simulink model "StFilteringLab"  (Simulink 7.6)
settings: Solver=VariableStepDiscrete  SolverMode=SingleTasking  StartTime=0.0  StopTime=4096*FirSamplingPeriod  RelTol=1e-3
PreLoadFcn:
  | clc
  | clear
  | close all
  | FilterOrder = 34;
  | InputBitWidth = 12;
  | CoefBitWidth = 14;
  | coef_max = 2^(CoefBitWidth - 1) - 1;
  | coef_min = -2^(CoefBitWidth - 1);
  | LowPassFreqBand = [0 0.001045 0.0015 1];
  | LowPassMagnBand = [1 0.975 0.00001 0.00001];
  | 
  | FlCoef_org = firls(FilterOrder,LowPassFreqBand,LowPassMagnBand);
  | w=blackman(FilterOrder + 1);
  | FlCoef_win = FlCoef_org .* w';
  | FlCoef = FlCoef_win;
  | ScalingFactor = max(coef_max/max(FlCoef), coef_min/min(FlCoef));
  | 
  | FpCoef = fix(ScalingFactor * FlCoef);
  | 
  | plot(FpCoef,'o');
  | title('Coefficient Value');
  | ImpulseData = zeros(1,1000);
  | ImpulseData(1) = 100;
  | h = conv(ImpulseData,FpCoef);
  | fftplot(h);
  | title('Frequency response');
  | FirSamplingPeriod=1;
InitFcn:
  | %% DSPBuilder Start
  | alt_dspbuilder_update_model(bdroot)
  | %% DSPBuilder End
StopFcn:
  | plot_fft(adder_result_sim, 'Frequency Response - Unfiltered Data', 8e7)
  |  plot_fft(fir_result_sim, 'Frequency Response - Filtered Data', 8e7)
values from neighbouring files (symbols this model uses):
  data = data(1:N)    [fftplot.m]
undefined symbols (not defined in the file or in its folder): filter_lib, lp_filter, Pin_AB15, Pin_AB6, Pin_AC14, Pin_AC19, Pin_AD14, Pin_AD18, Pin_AE3, Pin_AF25, Pin_AG23, Pin_G20, Pin_G3, Pin_G4, Pin_H3, Pin_H4, Pin_J5, Pin_J6, Pin_K1, Pin_K2, Pin_L1, Pin_L2, Pin_L3, Pin_L4, Pin_M7, Pin_M8, Pin_N3, Pin_N4, Pin_P1, Pin_P2, Pin_R3, Pin_R4, Pin_R6, Pin_R7, Pin_T3, Pin_T4, Pin_V3, Pin_V4, sin_gen
libraries: allblocks_alteradspbuilder2 x68, Cyclone_III_EP3C120_alteradspbuilder2 x5
settings Model: Creator=akarapet  LastModifiedBy=akarapet
settings DataIOCC: SignalLoggingName=sigsOut
settings OptimizationCC: InlineInvariantSignals=on  InitFltsAndDblsToZero=on
settings DebuggingCC: SaveWithParameterizedLinksMsg=none  SignalResolutionControl=TryResolveAllWithWarning  SolverPrmCheckMsg=none  MultiTaskDSMMsg=warning  MultiTaskCondExecSysMsg=none  StrictBusMsg=None
settings HardwareCC: TargetUnknown=on
settings RTWCC: IncludeERTFirstTime=on
settings GRTTargetCC: TargetFcnLib=ansi_tfl_tmw.mat

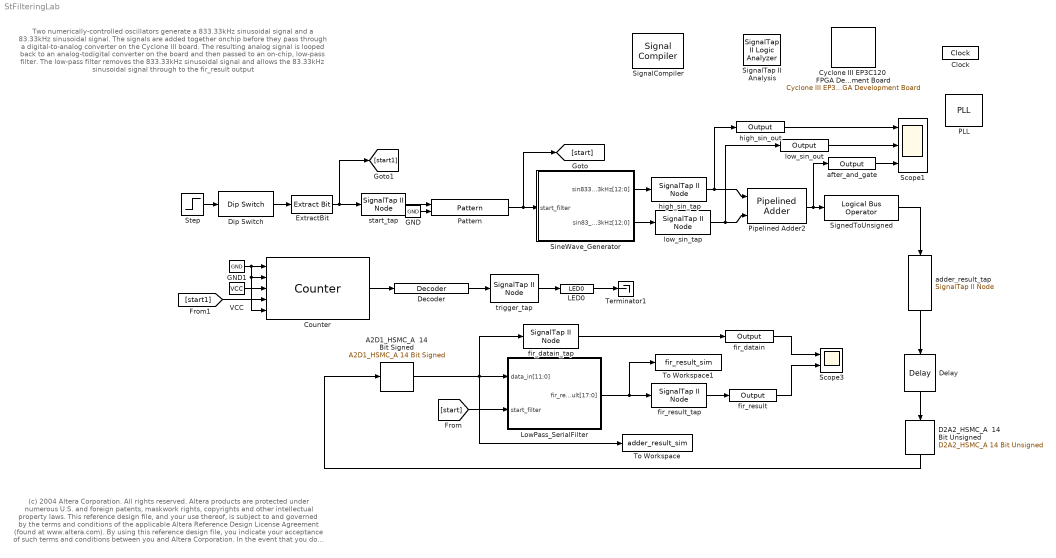
== system StFilteringLab ==
  note: (c) 2004 Altera Corporation. All rights reserved.  Altera products are protected under numerous U.S. and foreign patents, maskwork rights, copyrights and other intellectual property laws.
      | This reference design file, and your use thereof, is subject to and governed by the terms and conditions of the applicable Altera Reference Design License Agreement (found at www.altera.com).
      | By using this reference design file, you indicate your acceptance of such terms and conditions between you and Altera Corporation.
      | In the event that you do not agree with such terms and conditions, you may not use the reference design file and please promptly destroy any copies you have made.
      | This reference design file being provided on an "as-is" basis and as an accommodation and therefore all warranties, representations or guarantees of any kind (whether express, implied or statutory)
      | including, without limitation, warranties of merchantability, non-infringement, or fitness for a particular purpose, are specifically disclaimed.
      | By making this reference design file available, Altera expressly does not recommend, suggest or require that this reference design file be used in combination with any other product not provided by Altera
  note: Two numerically-controlled oscillators generate a 833.33kHz  sinusoidal
      | signal and a 83.33kHz sinusoidal signal. The signals are added together onchip
      | before they pass through a digital-to-analog converter on the Cyclone III board.
      | The resulting analog signal is looped back to an analog-todigital
      | converter on the board and then passed to an on-chip, low-pass
      | filter. The low-pass filter removes the 833.33kHz sinusoidal signal and
      | allows the 83.33kHz sinusoidal signal
      | through to the fir_result output
  A2D1_HSMC_A  14 Bit Signed : Cyclone_III_EP3C120_alteradspbuilder2/A2D1_HSMC_A 14 Bit Signed  iofile=/data/akarapet/qshell_linux64_test/p4/dsp_builder/dsp_builder2/Documentation/DesignExamples/Demos/Filters/FilteringLab/Stap/tb_StFilteringLab/StFilteringLab_A2D1%5FHSMC%5FA+%0A14+Bit+Signed.salt  externalType=Inferred  SpecifyClock=off  location=Pin_P1,Pin_P2,Pin_M7,Pin_M8,Pin_R4,Pin_R3,Pin_T3,Pin_T4,Pin_V3,Pin_V4,Pin_R6,Pin_R7,Pin_AE3,Pin_AB6
  Clock : allblocks_alteradspbuilder2/Clock  ClockPeriod=10  ClockPeriodUnit=ns  SampleTime=1  ResetLatency=0  ResetRegisterCascadeDepth=0  SimulationStartCycle=5  PhaseOffset=0  Reset=aclr  ResetType=Active Low  Export=off
  Counter : allblocks_alteradspbuilder2/Counter  BusType=Signed Integer  bwl=13  bwr=0  use_modulo=on  modulo=2^12 - 1  SpecifyClock=off  direction=Use Direction Port (updown)  use_sload=on  use_sset=off  svalue=1  use_clk_ena=on  use_ena=off  use_sclr=on  pipeline_display=1
  Cyclone III EP3C120  FPGA Development Board : Cyclone_III_EP3C120_alteradspbuilder2/Cyclone III EP3C120 FPGA Development Board  ClockPinIn=Pin_AH15  GlobalResetPin=Pin_T21  device=EP3C120F780C7
  D2A2_HSMC_A  14 Bit Unsigned : Cyclone_III_EP3C120_alteradspbuilder2/D2A2_HSMC_A 14 Bit Unsigned  iofile=/data/akarapet/qshell_linux64_test/p4/dsp_builder/dsp_builder2/Documentation/DesignExamples/Demos/Filters/FilteringLab/Stap/tb_StFilteringLab/StFilteringLab_D2A2%5FHSMC%5FA+%0A14+Bit+Unsigned.capture  externalType=Inferred  location=Pin_G3,Pin_G4,Pin_H3,Pin_H4,Pin_J5,Pin_J6,Pin_K1,Pin_K2,Pin_L1,Pin_L2,Pin_L3,Pin_L4,Pin_N3,Pin_N4
  Decoder : allblocks_alteradspbuilder2/Decoder  BusType=Signed Integer  bwl=13  bwr=0  registered=off  pipeline_display=0  value=1000
  Delay : allblocks_alteradspbuilder2/Delay  pipeline=1  pipeline_display=1  ClockPhase=1  use_ena=off  use_sclr=off  allowFloatingPointOverride=on  logOutputs=off  logFile=/data/akarapet/qshell_linux64_test/p4/dsp_builder/dsp_builder2/Documentation/DesignExamples/Demos/Filters/FilteringLab/Stap/tb_StFilteringLab/StFilteringLab_Delay.fixedpointlog  use_init=off  reset_value=1
  Dip Switch : Cyclone_III_EP3C120_alteradspbuilder2/Dip Switch  iofile=/data/akarapet/qshell_linux64_test/p4/dsp_builder/dsp_builder2/Documentation/DesignExamples/Demos/Filters/FilteringLab/Stap/tb_StFilteringLab/StFilteringLab_Dip+Switch.salt  externalType=Inferred  SpecifyClock=off  location=Pin_AC14,Pin_AD18,Pin_AG23,Pin_AC19,Pin_AD14,Pin_G20,Pin_AB15,Pin_AF25
  ExtractBit : allblocks_alteradspbuilder2/Extract Bit  BusType=Signed Fractional  bwl=8  bwr=0  bitToSelect=0  pipeline_display=0
  GND : allblocks_alteradspbuilder2/GND  SpecifyClock=off
  GND1 : allblocks_alteradspbuilder2/GND  SpecifyClock=off
  LED0 : Cyclone_III_EP3C120_alteradspbuilder2/LED0  iofile=/data/akarapet/qshell_linux64_test/p4/dsp_builder/dsp_builder2/Documentation/DesignExamples/Demos/Filters/FilteringLab/Stap/tb_StFilteringLab/StFilteringLab_LED0.capture  externalType=Inferred  location=Pin_AD15
  LowPass_SerialFilter : Subsystem  AncestorBlock=filter_lib/lp_filter
      mask Type: SubSystem AlteraBlockSet
  PLL : allblocks_alteradspbuilder2/PLL  clock_mult=[1, 1, 1, 1, 1, 1, 1, 1, 1]  clock_divide=[1, 1, 1, 1, 1, 1, 1, 1, 1]  clock_export=[1, 1, 1, 0, 0, 0, 0, 0, 0]  num_clocks=3  input_clock=Clock  use_base_clock=on
  Pattern : allblocks_alteradspbuilder2/Pattern  Sequence=100000000000  SpecifyClock=off  use_ena=on  use_sclr=on
  Pipelined Adder2 : allblocks_alteradspbuilder2/Pipelined Adder  BusType=Signed Integer  bwl=14  bwr=0  pipeline=1  pipeline_display=1  AddSubDirection=ADD  use_cin=off  use_ovl=off  use_addsub=off  use_ena=off  use_aclr=off  or_aclr_inputs=on
  Scope1 : Scope  NumInputPorts=3
      settings: YMin=-5~-5~-5  YMax=5~5~5  SaveName=ScopeData3
  Scope3 : Scope  NumInputPorts=2
      settings: YMin=-5~-5  YMax=5~5
  SignalCompiler : allblocks_alteradspbuilder2/Signal Compiler  DeviceFamily=Cyclone III  DeviceName=EP3C120F780C7  EnableSignalTap=on  SignalTapDepth=2048  UseBoardBlock=on  StpUseDefaultClock=on  StpClock=Clock  ExportDir=<binary blob, 123 chars, not shown>
  SignalTap II Analysis : allblocks_alteradspbuilder2/SignalTap II Logic Analyzer
  SignedToUnsigned : allblocks_alteradspbuilder2/Logical Bus Operator  BusType=Signed Fractional  bwl=14  bwr=0  LogicalOp_text=XOR  mask_value_num=8192  shift_amount=3  force_sign_ext=off  pipeline_display=0
  SineWave_Generator : Subsystem  AncestorBlock=filter_lib/sin_gen
      mask Type: SubSystem AlteraBlockSet
  Step : Step  SampleTime=FirSamplingPeriod
  Terminator1 : Terminator
  To Workspace : ToWorkspace  VariableName=adder_result_sim  SampleTime=FirSamplingPeriod  SaveFormat=Array
  To Workspace1 : ToWorkspace  VariableName=fir_result_sim  SampleTime=FirSamplingPeriod  SaveFormat=Array
  VCC : allblocks_alteradspbuilder2/VCC  SpecifyClock=off
  adder_result_tap : allblocks_alteradspbuilder2/SignalTap II Node  id=0
  after_and_gate : allblocks_alteradspbuilder2/Output  iofile=/data/akarapet/qshell_linux64_test/p4/dsp_builder/dsp_builder2/Documentation/DesignExamples/Demos/Filters/FilteringLab/Stap/tb_StFilteringLab/StFilteringLab_after%5Fand%5Fgate.capture  BusType=Signed Integer  bwl=14  bwr=0  externalType=Inferred  PORTTYPE=Output  allowFloatingPointOverride=on  logOutputs=off
  fir_datain : allblocks_alteradspbuilder2/Output  iofile=/data/akarapet/qshell_linux64_test/p4/dsp_builder/dsp_builder2/Documentation/DesignExamples/Demos/Filters/FilteringLab/Stap/tb_StFilteringLab/StFilteringLab_fir%5Fdatain.capture  BusType=Signed Integer  bwl=12  bwr=0  externalType=Inferred  PORTTYPE=Output  allowFloatingPointOverride=on  logOutputs=off
  fir_datain_tap : allblocks_alteradspbuilder2/SignalTap II Node  id=1
  fir_result : allblocks_alteradspbuilder2/Output  iofile=/data/akarapet/qshell_linux64_test/p4/dsp_builder/dsp_builder2/Documentation/DesignExamples/Demos/Filters/FilteringLab/Stap/tb_StFilteringLab/StFilteringLab_fir%5Fresult.capture  BusType=Signed Integer  bwl=18  bwr=0  externalType=Inferred  PORTTYPE=Output  allowFloatingPointOverride=on  logOutputs=off
  fir_result_tap : allblocks_alteradspbuilder2/SignalTap II Node  id=2
  high_sin_out : allblocks_alteradspbuilder2/Output  iofile=/data/akarapet/qshell_linux64_test/p4/dsp_builder/dsp_builder2/Documentation/DesignExamples/Demos/Filters/FilteringLab/Stap/tb_StFilteringLab/StFilteringLab_high%5Fsin%5Fout.capture  BusType=Signed Integer  bwl=13  bwr=0  externalType=Inferred  PORTTYPE=Output  allowFloatingPointOverride=on  logOutputs=off
  high_sin_tap : allblocks_alteradspbuilder2/SignalTap II Node  id=3
  low_sin_out : allblocks_alteradspbuilder2/Output  iofile=/data/akarapet/qshell_linux64_test/p4/dsp_builder/dsp_builder2/Documentation/DesignExamples/Demos/Filters/FilteringLab/Stap/tb_StFilteringLab/StFilteringLab_low%5Fsin%5Fout.capture  BusType=Signed Integer  bwl=13  bwr=0  externalType=Inferred  PORTTYPE=Output  allowFloatingPointOverride=on  logOutputs=off
  low_sin_tap : allblocks_alteradspbuilder2/SignalTap II Node  id=4
  start_tap : allblocks_alteradspbuilder2/SignalTap II Node  id=5
  trigger_tap : allblocks_alteradspbuilder2/SignalTap II Node  id=6
  wires:
  LowPass_SerialFilter/1(fir_result[17:0]) -> To Workspace1/1, fir_result_tap/1
  ExtractBit/1 -> start_tap/1, [start1]
  Step/1 -> Dip Switch/1
  GND/1 -> Pattern/2
  A2D1_HSMC_A  14 Bit Signed/1 -> LowPass_SerialFilter/1(data_in[11:0]), To Workspace/1, fir_datain_tap/1
  [start] -> LowPass_SerialFilter/2(start_filter)
  SignedToUnsigned/1 -> adder_result_tap/1
  SineWave_Generator/1(sin833_33kHz[12:0]) -> high_sin_tap/1
  SineWave_Generator/2(sin83_33kHz[12:0]) -> low_sin_tap/1
  adder_result_tap/1 -> Delay/1
  fir_result_tap/1 -> fir_result/1
  fir_result/1 -> Scope3/2
  Dip Switch/1 -> ExtractBit/1
  start_tap/1 -> Pattern/1
  high_sin_tap/1 -> Pipelined Adder2/1, high_sin_out/1
  low_sin_tap/1 -> Pipelined Adder2/2, low_sin_out/1
  [start1] -> Counter/4
  Decoder/1 -> trigger_tap/1
  Counter/1 -> Decoder/1
  trigger_tap/1 -> LED0/1
  VCC/1 -> Counter/3
  fir_datain_tap/1 -> fir_datain/1
  fir_datain/1 -> Scope3/1
  Delay/1 -> D2A2_HSMC_A  14 Bit Unsigned/1
  Pipelined Adder2/1 -> SignedToUnsigned/1, after_and_gate/1
  GND1/1 -> Counter/1, Counter/2, Counter/5
  Pattern/1 -> [start], SineWave_Generator/1(start_filter)
  high_sin_out/1 -> Scope1/1
  low_sin_out/1 -> Scope1/2
  after_and_gate/1 -> Scope1/3
  D2A2_HSMC_A  14 Bit Unsigned/1 -> A2D1_HSMC_A  14 Bit Signed/1
  LED0/1 -> Terminator1/1

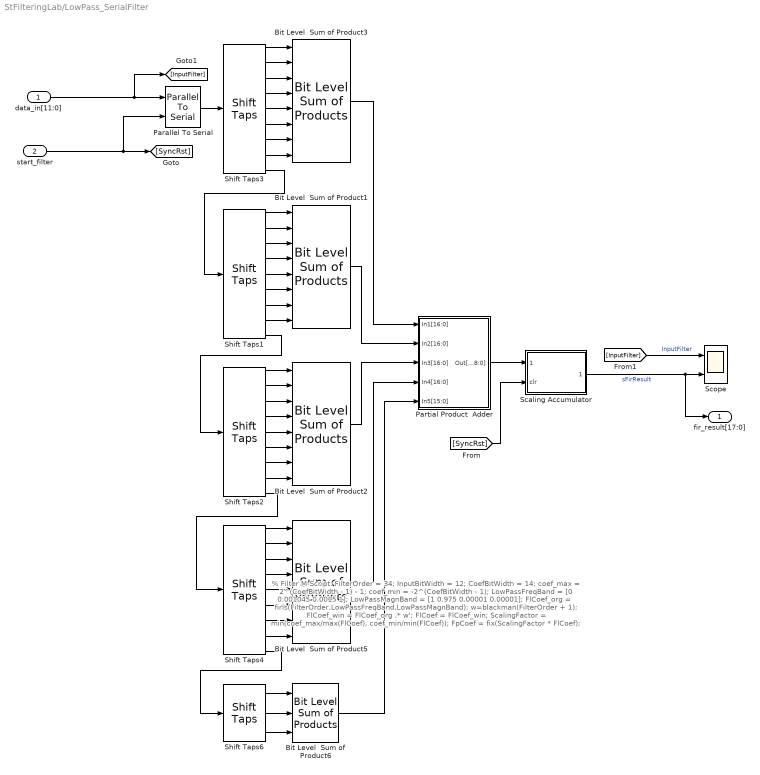
== system StFilteringLab/LowPass_SerialFilter ==
  note: % Filter M-Script:
      | FilterOrder = 34;
      | InputBitWidth = 12;
      | CoefBitWidth = 14;
      | coef_max = 2^(CoefBitWidth - 1) - 1;
      | coef_min = -2^(CoefBitWidth - 1);
      | LowPassFreqBand = [0 0.001045 0.0015 1];
      | LowPassMagnBand = [1 0.975 0.00001 0.00001];
      | FlCoef_org = firls(FilterOrder,LowPassFreqBand,LowPassMagnBand);
      | w=blackman(FilterOrder + 1);
      | FlCoef_win = FlCoef_org .* w';
      | FlCoef = FlCoef_win;
      | ScalingFactor = min(coef_max/max(FlCoef), coef_min/min(FlCoef));
      | FpCoef = fix(ScalingFactor * FlCoef);
  data_in[11:0] : Inport
  start_filter : Inport  Port=2
  Bit Level  Sum of Product1 : allblocks_alteradspbuilder2/Bit Level Sum of Products  number_of_coefficients=8  BusType=Signed Integer  bwl=14  bwr=0  coefficients=[FpCoef(9:16)]  register_inputs=off  pipeline_display=0  use_ena=off  use_sclr=off  allowFloatingPointOverride=on  logOutputs=off  logFile=/data/akarapet/qshell_linux64_test/p4/dsp_builder/dsp_builder2/Documentation/DesignExamples/Demos/Filters/FilteringLab/Stap/tb_StFilteringLab/StFilteringLab_LowPass%5FSerialFilter_Bit+Level+%0ASum+of+Product1.fixedpointlog
  Bit Level  Sum of Product2 : allblocks_alteradspbuilder2/Bit Level Sum of Products  number_of_coefficients=8  BusType=Signed Integer  bwl=14  bwr=0  coefficients=[FpCoef(17:24)]  register_inputs=off  pipeline_display=0  use_ena=off  use_sclr=off  allowFloatingPointOverride=on  logOutputs=off  logFile=/data/akarapet/qshell_linux64_test/p4/dsp_builder/dsp_builder2/Documentation/DesignExamples/Demos/Filters/FilteringLab/Stap/tb_StFilteringLab/StFilteringLab_LowPass%5FSerialFilter_Bit+Level+%0ASum+of+Product2.fixedpointlog
  Bit Level  Sum of Product3 : allblocks_alteradspbuilder2/Bit Level Sum of Products  number_of_coefficients=8  BusType=Signed Integer  bwl=14  bwr=0  coefficients=[FpCoef(1:8)]  register_inputs=off  pipeline_display=0  use_ena=off  use_sclr=off  allowFloatingPointOverride=on  logOutputs=off  logFile=/data/akarapet/qshell_linux64_test/p4/dsp_builder/dsp_builder2/Documentation/DesignExamples/Demos/Filters/FilteringLab/Stap/tb_StFilteringLab/StFilteringLab_LowPass%5FSerialFilter_Bit+Level+%0ASum+of+Product3.fixedpointlog
  Bit Level  Sum of Product5 : allblocks_alteradspbuilder2/Bit Level Sum of Products  number_of_coefficients=8  BusType=Signed Integer  bwl=14  bwr=0  coefficients=[FpCoef(25:32)]  register_inputs=off  pipeline_display=0  use_ena=off  use_sclr=off  allowFloatingPointOverride=on  logOutputs=off  logFile=/data/akarapet/qshell_linux64_test/p4/dsp_builder/dsp_builder2/Documentation/DesignExamples/Demos/Filters/FilteringLab/Stap/tb_StFilteringLab/StFilteringLab_LowPass%5FSerialFilter_Bit+Level+%0ASum+of+Product5.fixedpointlog
  Bit Level  Sum of Product6 : allblocks_alteradspbuilder2/Bit Level Sum of Products  number_of_coefficients=3  BusType=Signed Integer  bwl=14  bwr=0  coefficients=[FpCoef(33:35)]  register_inputs=off  pipeline_display=0  use_ena=off  use_sclr=off  allowFloatingPointOverride=on  logOutputs=off  logFile=/data/akarapet/qshell_linux64_test/p4/dsp_builder/dsp_builder2/Documentation/DesignExamples/Demos/Filters/FilteringLab/Stap/tb_StFilteringLab/StFilteringLab_LowPass%5FSerialFilter_Bit+Level+%0ASum+of+Product6.fixedpointlog
  Parallel To Serial : allblocks_alteradspbuilder2/Parallel To Serial  BusType=Signed Integer  bwl=12  bwr=0  msbfirsttext=LSB First  msbfirst=0  repeatlastbit=on  use_ena=off  use_sclr=off
  Partial Product  Adder : Subsystem  AncestorBlock=ALTELINK/AltLab/HDL SubSystem
      mask Type: SubSystem AlteraBlockSet
  Scaling Accumulator : Subsystem  AncestorBlock=ALTELINK/AltLab/HDL SubSystem
      mask Type: SubSystem AlteraBlockSet
  Scope : Scope  NumInputPorts=2
      settings: YMin=-125~-25  YMax=125~25
  Shift Taps1 : allblocks_alteradspbuilder2/Shift Taps  number_of_taps=8  tap_distance=12  use_shiftout=on  use_ena=off  use_sclr=off  use_dedicated_circuitry=on  ram_type=AUTO  allowFloatingPointOverride=on  logOutputs=off  logFile=/data/akarapet/qshell_linux64_test/p4/dsp_builder/dsp_builder2/Documentation/DesignExamples/Demos/Filters/FilteringLab/Stap/tb_StFilteringLab/StFilteringLab_LowPass%5FSerialFilter_Shift+Taps1%3A%3At.fixedpointlog,/data/akarapet/qshell_linux64_test/p4/dsp_builder/dsp_builder2/Documentation/DesignExamples/Demos/Filters/FilteringLab/Stap/tb_StFilteringLab/StFilteringLab_LowPass%5FSerialFilter_Shift+Taps1%3A%3At.fixedpointlog,/data/akarapet/qshell_linux64_test/p4/dsp_builder/dsp_builder2/Documentation/DesignExamples/Demos/Filters/FilteringLab/Stap/tb_StFilteringLab/StFilteringLab_LowPass%5FSerialFilter_Shift+Taps1%3A%3At.fixedpointlog,/data/akarapet/qshell_linux64_test/p4/dsp_builder/dsp_builder2/Documentation/DesignExamples/Demos/Filters/FilteringLab/Stap/tb_StFilteringLab/StFilteringLab_LowPass%5FSerialFilter_Shift+Taps1%3A%3At.fixedpointlog,/data/akarapet/qshell_linux64_test/p4/dsp_builder/dsp_builder2/Documentation/DesignExamples/Demos/Filters/FilteringLab/Stap/tb_StFilteringLab/StFilteringLab_LowPass%5FSerialFilter_Shift+Taps1%3A%3At.fixedpointlog,/data/akarapet/qshell_linux64_test/p4/dsp_builder/dsp_builder2/Documentation/DesignExamples/Demos/Filters/FilteringLab/Stap/tb_StFilteringLab/StFilteringLab_LowPass%5FSerialFilter_Shift+Taps1%3A%3At.fixedpointlog,/data/akarapet/qshell_linux64_test/p4/dsp_builder/dsp_builder2/Documentation/DesignExamples/Demos/Filters/FilteringLab/Stap/tb_StFilteringLab/StFilteringLab_LowPass%5FSerialFilter_Shift+Taps1%3A%3At.fixedpointlog,/data/akarapet/qshell_linux64_test/p4/dsp_builder/dsp_builder2/Documentation/DesignExamples/Demos/Filters/FilteringLab/Stap/tb_StFilteringLab/StFilteringLab_LowPass%5FSerialFilter_Shift+Taps1%3A%3At.fixedpointlog,/data/akarapet/qshell_linux64_test/p4/dsp_builder/dsp_builder2/Documentation/DesignExamples/Demos/Filters/FilteringLab/Stap/tb_StFilteringLab/StFilteringLab_LowPass%5FSerialFilter_Shift+Taps1%3A%3Ashiftout.fixedpointlog,
  Shift Taps2 : allblocks_alteradspbuilder2/Shift Taps  number_of_taps=8  tap_distance=12  use_shiftout=on  use_ena=off  use_sclr=off  use_dedicated_circuitry=on  ram_type=AUTO  allowFloatingPointOverride=on  logOutputs=off  logFile=/data/akarapet/qshell_linux64_test/p4/dsp_builder/dsp_builder2/Documentation/DesignExamples/Demos/Filters/FilteringLab/Stap/tb_StFilteringLab/StFilteringLab_LowPass%5FSerialFilter_Shift+Taps2%3A%3At.fixedpointlog,/data/akarapet/qshell_linux64_test/p4/dsp_builder/dsp_builder2/Documentation/DesignExamples/Demos/Filters/FilteringLab/Stap/tb_StFilteringLab/StFilteringLab_LowPass%5FSerialFilter_Shift+Taps2%3A%3At.fixedpointlog,/data/akarapet/qshell_linux64_test/p4/dsp_builder/dsp_builder2/Documentation/DesignExamples/Demos/Filters/FilteringLab/Stap/tb_StFilteringLab/StFilteringLab_LowPass%5FSerialFilter_Shift+Taps2%3A%3At.fixedpointlog,/data/akarapet/qshell_linux64_test/p4/dsp_builder/dsp_builder2/Documentation/DesignExamples/Demos/Filters/FilteringLab/Stap/tb_StFilteringLab/StFilteringLab_LowPass%5FSerialFilter_Shift+Taps2%3A%3At.fixedpointlog,/data/akarapet/qshell_linux64_test/p4/dsp_builder/dsp_builder2/Documentation/DesignExamples/Demos/Filters/FilteringLab/Stap/tb_StFilteringLab/StFilteringLab_LowPass%5FSerialFilter_Shift+Taps2%3A%3At.fixedpointlog,/data/akarapet/qshell_linux64_test/p4/dsp_builder/dsp_builder2/Documentation/DesignExamples/Demos/Filters/FilteringLab/Stap/tb_StFilteringLab/StFilteringLab_LowPass%5FSerialFilter_Shift+Taps2%3A%3At.fixedpointlog,/data/akarapet/qshell_linux64_test/p4/dsp_builder/dsp_builder2/Documentation/DesignExamples/Demos/Filters/FilteringLab/Stap/tb_StFilteringLab/StFilteringLab_LowPass%5FSerialFilter_Shift+Taps2%3A%3At.fixedpointlog,/data/akarapet/qshell_linux64_test/p4/dsp_builder/dsp_builder2/Documentation/DesignExamples/Demos/Filters/FilteringLab/Stap/tb_StFilteringLab/StFilteringLab_LowPass%5FSerialFilter_Shift+Taps2%3A%3At.fixedpointlog,/data/akarapet/qshell_linux64_test/p4/dsp_builder/dsp_builder2/Documentation/DesignExamples/Demos/Filters/FilteringLab/Stap/tb_StFilteringLab/StFilteringLab_LowPass%5FSerialFilter_Shift+Taps2%3A%3Ashiftout.fixedpointlog,
  Shift Taps3 : allblocks_alteradspbuilder2/Shift Taps  number_of_taps=8  tap_distance=12  use_shiftout=on  use_ena=off  use_sclr=off  use_dedicated_circuitry=on  ram_type=AUTO  allowFloatingPointOverride=on  logOutputs=off  logFile=/data/akarapet/qshell_linux64_test/p4/dsp_builder/dsp_builder2/Documentation/DesignExamples/Demos/Filters/FilteringLab/Stap/tb_StFilteringLab/StFilteringLab_LowPass%5FSerialFilter_Shift+Taps3%3A%3At.fixedpointlog,/data/akarapet/qshell_linux64_test/p4/dsp_builder/dsp_builder2/Documentation/DesignExamples/Demos/Filters/FilteringLab/Stap/tb_StFilteringLab/StFilteringLab_LowPass%5FSerialFilter_Shift+Taps3%3A%3At.fixedpointlog,/data/akarapet/qshell_linux64_test/p4/dsp_builder/dsp_builder2/Documentation/DesignExamples/Demos/Filters/FilteringLab/Stap/tb_StFilteringLab/StFilteringLab_LowPass%5FSerialFilter_Shift+Taps3%3A%3At.fixedpointlog,/data/akarapet/qshell_linux64_test/p4/dsp_builder/dsp_builder2/Documentation/DesignExamples/Demos/Filters/FilteringLab/Stap/tb_StFilteringLab/StFilteringLab_LowPass%5FSerialFilter_Shift+Taps3%3A%3At.fixedpointlog,/data/akarapet/qshell_linux64_test/p4/dsp_builder/dsp_builder2/Documentation/DesignExamples/Demos/Filters/FilteringLab/Stap/tb_StFilteringLab/StFilteringLab_LowPass%5FSerialFilter_Shift+Taps3%3A%3At.fixedpointlog,/data/akarapet/qshell_linux64_test/p4/dsp_builder/dsp_builder2/Documentation/DesignExamples/Demos/Filters/FilteringLab/Stap/tb_StFilteringLab/StFilteringLab_LowPass%5FSerialFilter_Shift+Taps3%3A%3At.fixedpointlog,/data/akarapet/qshell_linux64_test/p4/dsp_builder/dsp_builder2/Documentation/DesignExamples/Demos/Filters/FilteringLab/Stap/tb_StFilteringLab/StFilteringLab_LowPass%5FSerialFilter_Shift+Taps3%3A%3At.fixedpointlog,/data/akarapet/qshell_linux64_test/p4/dsp_builder/dsp_builder2/Documentation/DesignExamples/Demos/Filters/FilteringLab/Stap/tb_StFilteringLab/StFilteringLab_LowPass%5FSerialFilter_Shift+Taps3%3A%3At.fixedpointlog,/data/akarapet/qshell_linux64_test/p4/dsp_builder/dsp_builder2/Documentation/DesignExamples/Demos/Filters/FilteringLab/Stap/tb_StFilteringLab/StFilteringLab_LowPass%5FSerialFilter_Shift+Taps3%3A%3Ashiftout.fixedpointlog,
  Shift Taps4 : allblocks_alteradspbuilder2/Shift Taps  number_of_taps=8  tap_distance=12  use_shiftout=on  use_ena=off  use_sclr=off  use_dedicated_circuitry=on  ram_type=AUTO  allowFloatingPointOverride=on  logOutputs=off  logFile=/data/akarapet/qshell_linux64_test/p4/dsp_builder/dsp_builder2/Documentation/DesignExamples/Demos/Filters/FilteringLab/Stap/tb_StFilteringLab/StFilteringLab_LowPass%5FSerialFilter_Shift+Taps4%3A%3At.fixedpointlog,/data/akarapet/qshell_linux64_test/p4/dsp_builder/dsp_builder2/Documentation/DesignExamples/Demos/Filters/FilteringLab/Stap/tb_StFilteringLab/StFilteringLab_LowPass%5FSerialFilter_Shift+Taps4%3A%3At.fixedpointlog,/data/akarapet/qshell_linux64_test/p4/dsp_builder/dsp_builder2/Documentation/DesignExamples/Demos/Filters/FilteringLab/Stap/tb_StFilteringLab/StFilteringLab_LowPass%5FSerialFilter_Shift+Taps4%3A%3At.fixedpointlog,/data/akarapet/qshell_linux64_test/p4/dsp_builder/dsp_builder2/Documentation/DesignExamples/Demos/Filters/FilteringLab/Stap/tb_StFilteringLab/StFilteringLab_LowPass%5FSerialFilter_Shift+Taps4%3A%3At.fixedpointlog,/data/akarapet/qshell_linux64_test/p4/dsp_builder/dsp_builder2/Documentation/DesignExamples/Demos/Filters/FilteringLab/Stap/tb_StFilteringLab/StFilteringLab_LowPass%5FSerialFilter_Shift+Taps4%3A%3At.fixedpointlog,/data/akarapet/qshell_linux64_test/p4/dsp_builder/dsp_builder2/Documentation/DesignExamples/Demos/Filters/FilteringLab/Stap/tb_StFilteringLab/StFilteringLab_LowPass%5FSerialFilter_Shift+Taps4%3A%3At.fixedpointlog,/data/akarapet/qshell_linux64_test/p4/dsp_builder/dsp_builder2/Documentation/DesignExamples/Demos/Filters/FilteringLab/Stap/tb_StFilteringLab/StFilteringLab_LowPass%5FSerialFilter_Shift+Taps4%3A%3At.fixedpointlog,/data/akarapet/qshell_linux64_test/p4/dsp_builder/dsp_builder2/Documentation/DesignExamples/Demos/Filters/FilteringLab/Stap/tb_StFilteringLab/StFilteringLab_LowPass%5FSerialFilter_Shift+Taps4%3A%3At.fixedpointlog,/data/akarapet/qshell_linux64_test/p4/dsp_builder/dsp_builder2/Documentation/DesignExamples/Demos/Filters/FilteringLab/Stap/tb_StFilteringLab/StFilteringLab_LowPass%5FSerialFilter_Shift+Taps4%3A%3Ashiftout.fixedpointlog,
  Shift Taps6 : allblocks_alteradspbuilder2/Shift Taps  number_of_taps=3  tap_distance=12  use_shiftout=off  use_ena=off  use_sclr=off  use_dedicated_circuitry=on  ram_type=AUTO  allowFloatingPointOverride=on  logOutputs=off  logFile=/data/akarapet/qshell_linux64_test/p4/dsp_builder/dsp_builder2/Documentation/DesignExamples/Demos/Filters/FilteringLab/Stap/tb_StFilteringLab/StFilteringLab_LowPass%5FSerialFilter_Shift+Taps6%3A%3At.fixedpointlog,/data/akarapet/qshell_linux64_test/p4/dsp_builder/dsp_builder2/Documentation/DesignExamples/Demos/Filters/FilteringLab/Stap/tb_StFilteringLab/StFilteringLab_LowPass%5FSerialFilter_Shift+Taps6%3A%3At.fixedpointlog,/data/akarapet/qshell_linux64_test/p4/dsp_builder/dsp_builder2/Documentation/DesignExamples/Demos/Filters/FilteringLab/Stap/tb_StFilteringLab/StFilteringLab_LowPass%5FSerialFilter_Shift+Taps6%3A%3At.fixedpointlog,
  fir_result[17:0] : Outport
  wires:
  Bit Level  Sum of Product6/1 -> Partial Product  Adder/5(In5[15:0])
  Bit Level  Sum of Product5/1 -> Partial Product  Adder/4(In4[16:0])
  Bit Level  Sum of Product2/1 -> Partial Product  Adder/3(In3[16:0])
  Bit Level  Sum of Product1/1 -> Partial Product  Adder/2(In2[16:0])
  Bit Level  Sum of Product3/1 -> Partial Product  Adder/1(In1[16:0])
  Shift Taps4/8 -> Bit Level  Sum of Product5/8
  Shift Taps4/7 -> Bit Level  Sum of Product5/7
  Shift Taps4/6 -> Bit Level  Sum of Product5/6
  Shift Taps4/5 -> Bit Level  Sum of Product5/5
  Shift Taps4/4 -> Bit Level  Sum of Product5/4
  Shift Taps4/3 -> Bit Level  Sum of Product5/3
  Shift Taps4/2 -> Bit Level  Sum of Product5/2
  Shift Taps4/1 -> Bit Level  Sum of Product5/1
  Shift Taps3/9 -> Shift Taps1/1
  Shift Taps3/8 -> Bit Level  Sum of Product3/8
  Shift Taps3/7 -> Bit Level  Sum of Product3/7
  Shift Taps3/6 -> Bit Level  Sum of Product3/6
  Shift Taps3/5 -> Bit Level  Sum of Product3/5
  Shift Taps3/4 -> Bit Level  Sum of Product3/4
  Shift Taps3/3 -> Bit Level  Sum of Product3/3
  Shift Taps3/2 -> Bit Level  Sum of Product3/2
  Shift Taps3/1 -> Bit Level  Sum of Product3/1
  Scaling Accumulator/1(Out[17:0]) -> fir_result[17:0]/1, Scope/2  "sFirResult"
  [InputFilter] -> Scope/1  "InputFilter"
  data_in[11:0]/1 -> Parallel To Serial/1, [InputFilter]
  Shift Taps2/9 -> Shift Taps4/1
  Shift Taps4/9 -> Shift Taps6/1
  Shift Taps6/3 -> Bit Level  Sum of Product6/3
  Shift Taps6/2 -> Bit Level  Sum of Product6/2
  Shift Taps6/1 -> Bit Level  Sum of Product6/1
  Partial Product  Adder/1(Out[18:0]) -> Scaling Accumulator/1(In[18:0])
  Parallel To Serial/1 -> Shift Taps3/1
  Shift Taps1/9 -> Shift Taps2/1
  Shift Taps2/8 -> Bit Level  Sum of Product2/8
  Shift Taps2/7 -> Bit Level  Sum of Product2/7
  Shift Taps2/6 -> Bit Level  Sum of Product2/6
  Shift Taps2/5 -> Bit Level  Sum of Product2/5
  Shift Taps2/4 -> Bit Level  Sum of Product2/4
  Shift Taps2/3 -> Bit Level  Sum of Product2/3
  Shift Taps2/2 -> Bit Level  Sum of Product2/2
  Shift Taps2/1 -> Bit Level  Sum of Product2/1
  Shift Taps1/8 -> Bit Level  Sum of Product1/8
  Shift Taps1/7 -> Bit Level  Sum of Product1/7
  Shift Taps1/6 -> Bit Level  Sum of Product1/6
  Shift Taps1/5 -> Bit Level  Sum of Product1/5
  Shift Taps1/4 -> Bit Level  Sum of Product1/4
  Shift Taps1/3 -> Bit Level  Sum of Product1/3
  Shift Taps1/2 -> Bit Level  Sum of Product1/2
  Shift Taps1/1 -> Bit Level  Sum of Product1/1
  start_filter/1 -> [SyncRst], Parallel To Serial/2
  [SyncRst] -> Scaling Accumulator/2(clr)

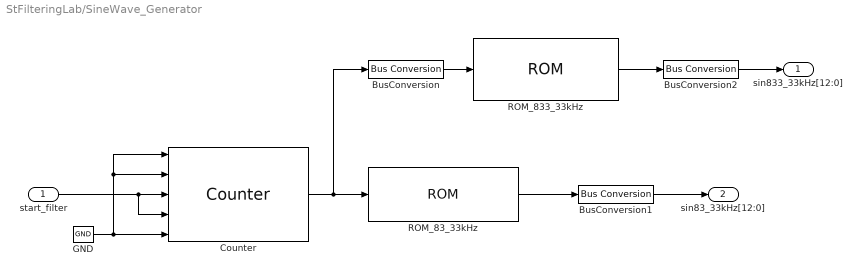
== system StFilteringLab/SineWave_Generator ==
  start_filter : Inport
  BusConversion : allblocks_alteradspbuilder2/Bus Conversion  BusType=Unsigned Integer  ibwl=7  ibwr=0  bwl=3  bwr=0  bitToConnectToOutputLSB=0  round=off  saturate=off  pipeline_display=0
  BusConversion1 : allblocks_alteradspbuilder2/Bus Conversion  BusType=Signed Integer  ibwl=16  ibwr=0  bwl=13  bwr=0  bitToConnectToOutputLSB=0  round=off  saturate=off  pipeline_display=0
  BusConversion2 : allblocks_alteradspbuilder2/Bus Conversion  BusType=Signed Integer  ibwl=16  ibwr=0  bwl=13  bwr=0  bitToConnectToOutputLSB=0  round=off  saturate=off  pipeline_display=0
  Counter : allblocks_alteradspbuilder2/Counter  BusType=Unsigned Integer  bwl=7  bwr=0  use_modulo=on  modulo=80  SpecifyClock=off  direction=Use Direction Port (updown)  use_sload=on  use_sset=off  svalue=1  use_clk_ena=on  use_ena=off  use_sclr=on  pipeline_display=1
  GND : allblocks_alteradspbuilder2/GND  SpecifyClock=off
  ROM_833_33kHz : allblocks_alteradspbuilder2/ROM  numwords=2^(16)  BusType=Signed Integer  bwl=16  bwr=0  memory_type=AUTO  ram_type=ROM  initialization=From HEX file  init_file=sin_833kHz.hex  init_array=[0:1:15]  register_outputs=off  use_ena=off  ClockPhase=1  pipeline_display=1  allowFloatingPointOverride=on  logOutputs=off  logFile=/data/akarapet/qshell_linux64_test/p4/dsp_builder/dsp_builder2/Documentation/DesignExamples/Demos/Filters/FilteringLab/Stap/tb_StFilteringLab/StFilteringLab_SineWave%5FGenerator_ROM%5F833%5F33kHz.fixedpointlog  enable_runtime_mod=off  instance_name=AAAA
  ROM_83_33kHz : allblocks_alteradspbuilder2/ROM  numwords=2^(16)  BusType=Signed Integer  bwl=16  bwr=0  memory_type=AUTO  ram_type=ROM  initialization=From HEX file  init_file=sin_83kHz.hex  init_array=[0:1:15]  register_outputs=off  use_ena=off  ClockPhase=1  pipeline_display=1  allowFloatingPointOverride=on  logOutputs=off  logFile=/data/akarapet/qshell_linux64_test/p4/dsp_builder/dsp_builder2/Documentation/DesignExamples/Demos/Filters/FilteringLab/Stap/tb_StFilteringLab/StFilteringLab_SineWave%5FGenerator_ROM%5F83%5F33kHz.fixedpointlog  enable_runtime_mod=off  instance_name=AAAA
  sin833_33kHz[12:0] : Outport
  sin83_33kHz[12:0] : Outport  Port=2
  wires:
  BusConversion1/1 -> sin83_33kHz[12:0]/1
  ROM_83_33kHz/1 -> BusConversion1/1
  BusConversion2/1 -> sin833_33kHz[12:0]/1
  ROM_833_33kHz/1 -> BusConversion2/1
  Counter/1 -> ROM_83_33kHz/1, BusConversion/1
  start_filter/1 -> Counter/4, Counter/3
  BusConversion/1 -> ROM_833_33kHz/1
  GND/1 -> Counter/1, Counter/2, Counter/5

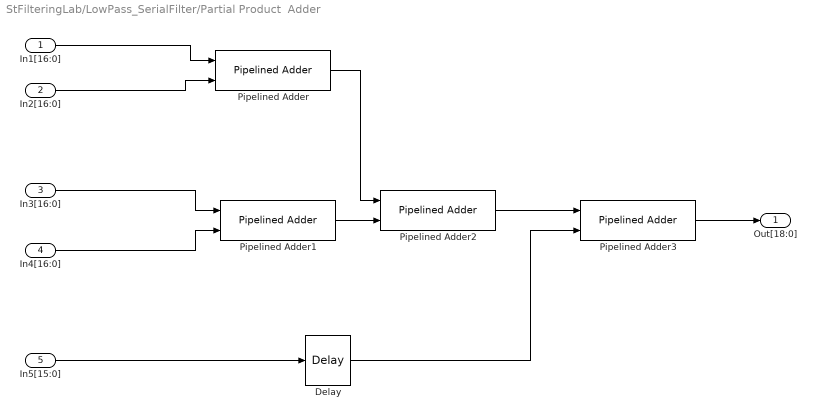
== system StFilteringLab/LowPass_SerialFilter/Partial Product  Adder ==
  In1[16:0] : Inport
  In2[16:0] : Inport  Port=2
  In3[16:0] : Inport  Port=3
  In4[16:0] : Inport  Port=4
  In5[15:0] : Inport  Port=5
  Delay : allblocks_alteradspbuilder2/Delay  pipeline=3  pipeline_display=3  ClockPhase=1  use_ena=off  use_sclr=off  allowFloatingPointOverride=on  logOutputs=off  logFile=/data/akarapet/qshell_linux64_test/p4/dsp_builder/dsp_builder2/Documentation/DesignExamples/Demos/Filters/FilteringLab/Stap/tb_StFilteringLab/StFilteringLab_LowPass%5FSerialFilter_Partial+Product+%0AAdder_Delay.fixedpointlog  use_init=off  reset_value=1
  Pipelined Adder : allblocks_alteradspbuilder2/Pipelined Adder  BusType=Signed Integer  bwl=18  bwr=0  pipeline=2  pipeline_display=2  AddSubDirection=ADD  use_cin=off  use_ovl=off  use_addsub=off  use_ena=off  use_aclr=off  or_aclr_inputs=on
  Pipelined Adder1 : allblocks_alteradspbuilder2/Pipelined Adder  BusType=Signed Integer  bwl=18  bwr=0  pipeline=2  pipeline_display=2  AddSubDirection=ADD  use_cin=off  use_ovl=off  use_addsub=off  use_ena=off  use_aclr=off  or_aclr_inputs=on
  Pipelined Adder2 : allblocks_alteradspbuilder2/Pipelined Adder  BusType=Signed Integer  bwl=19  bwr=0  pipeline=1  pipeline_display=1  AddSubDirection=ADD  use_cin=off  use_ovl=off  use_addsub=off  use_ena=off  use_aclr=off  or_aclr_inputs=on
  Pipelined Adder3 : allblocks_alteradspbuilder2/Pipelined Adder  BusType=Signed Integer  bwl=19  bwr=0  pipeline=1  pipeline_display=1  AddSubDirection=ADD  use_cin=off  use_ovl=off  use_addsub=off  use_ena=off  use_aclr=off  or_aclr_inputs=on
  Out[18:0] : Outport
  wires:
  Delay/1 -> Pipelined Adder3/2
  In5[15:0]/1 -> Delay/1
  Pipelined Adder2/1 -> Pipelined Adder3/1
  Pipelined Adder3/1 -> Out[18:0]/1
  Pipelined Adder1/1 -> Pipelined Adder2/2
  Pipelined Adder/1 -> Pipelined Adder2/1
  In4[16:0]/1 -> Pipelined Adder1/2
  In3[16:0]/1 -> Pipelined Adder1/1
  In2[16:0]/1 -> Pipelined Adder/2
  In1[16:0]/1 -> Pipelined Adder/1

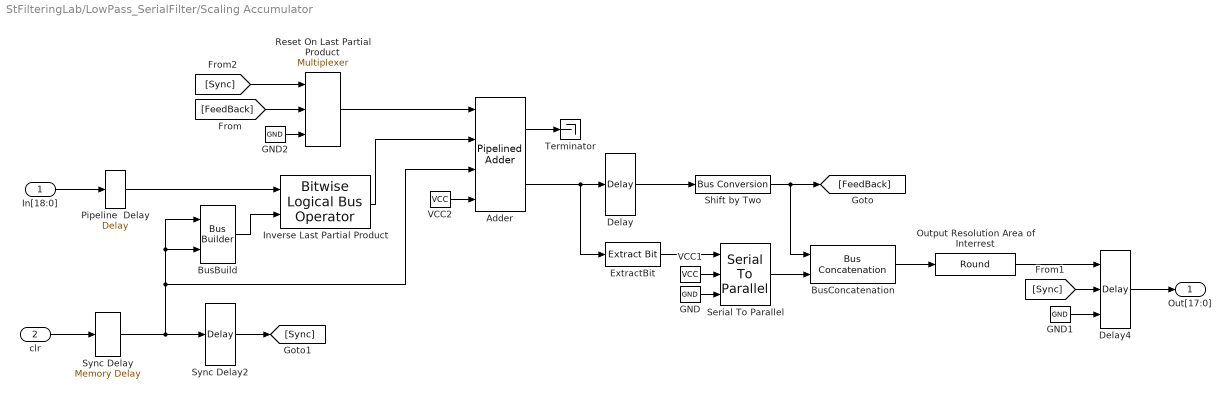
== system StFilteringLab/LowPass_SerialFilter/Scaling Accumulator ==
  In[18:0] : Inport
  clr : Inport  Port=2
  Adder : allblocks_alteradspbuilder2/Pipelined Adder  BusType=Signed Integer  bwl=20  bwr=0  pipeline=0  pipeline_display=0  AddSubDirection=ADD  use_cin=on  use_ovl=on  use_addsub=on  use_ena=on  use_aclr=on  or_aclr_inputs=on
  BusBuild : allblocks_alteradspbuilder2/Bus Builder  BusType=Signed Integer  bwl=2  bwr=0  pipeline_display=0
  BusConcatenation : allblocks_alteradspbuilder2/Bus Concatenation  isSigned=on  awidth=19  bwidth=12  pipeline_display=0
  Delay : allblocks_alteradspbuilder2/Delay  pipeline=1  pipeline_display=1  ClockPhase=1  use_ena=off  use_sclr=off  allowFloatingPointOverride=on  logOutputs=off  logFile=/data/akarapet/qshell_linux64_test/p4/dsp_builder/dsp_builder2/Documentation/DesignExamples/Demos/Filters/FilteringLab/Stap/tb_StFilteringLab/StFilteringLab_LowPass%5FSerialFilter_Scaling+Accumulator_Delay.fixedpointlog  use_init=off  reset_value=1
  Delay4 : allblocks_alteradspbuilder2/Delay  pipeline=1  pipeline_display=1  ClockPhase=1  use_ena=on  use_sclr=on  allowFloatingPointOverride=on  logOutputs=off  logFile=/data/akarapet/qshell_linux64_test/p4/dsp_builder/dsp_builder2/Documentation/DesignExamples/Demos/Filters/FilteringLab/Stap/tb_StFilteringLab/StFilteringLab_LowPass%5FSerialFilter_Scaling+Accumulator_Delay4.fixedpointlog  use_init=off  reset_value=1
  ExtractBit : allblocks_alteradspbuilder2/Extract Bit  BusType=Signed Fractional  bwl=21  bwr=0  bitToSelect=0  pipeline_display=0
  GND : allblocks_alteradspbuilder2/GND  SpecifyClock=off
  GND1 : allblocks_alteradspbuilder2/GND  SpecifyClock=off
  GND2 : allblocks_alteradspbuilder2/GND  SpecifyClock=off
  Inverse Last Partial Product : allblocks_alteradspbuilder2/Bitwise Logical Bus Operator  BusType=Signed Integer  bwl=19  bwr=0  LogicalOperator=XOR  pipeline_display=0
  Output Resolution Area of Interrest : allblocks_alteradspbuilder2/Round  BusType=Signed Integer  bwl=31  bwr=0  bitsToRemove=14  roundMode=ROUND_UP_SYM  userRoundMode=Round Away From Zero  pipeline=off  pipeline_display=0  use_ena=off  use_aclr=off
  Pipeline  Delay : allblocks_alteradspbuilder2/Delay  pipeline=1  pipeline_display=1  ClockPhase=1  use_ena=off  use_sclr=off  allowFloatingPointOverride=on  logOutputs=off  logFile=/data/akarapet/qshell_linux64_test/p4/dsp_builder/dsp_builder2/Documentation/DesignExamples/Demos/Filters/FilteringLab/Stap/tb_StFilteringLab/StFilteringLab_LowPass%5FSerialFilter_Scaling+Accumulator_Pipeline+%0ADelay.fixedpointlog  use_init=off  reset_value=1
  Reset On Last Partial Product : allblocks_alteradspbuilder2/Multiplexer  numInputs=2  pipeline=0  oneHot=off  pipeline_display=0  use_ena=off  use_aclr=off  allowFloatingPointOverride=on  logOutputs=off  logFile=/data/akarapet/qshell_linux64_test/p4/dsp_builder/dsp_builder2/Documentation/DesignExamples/Demos/Filters/FilteringLab/Stap/tb_StFilteringLab/StFilteringLab_LowPass%5FSerialFilter_Scaling+Accumulator_Reset+On%0ALast+Partial+Product.fixedpointlog
  Serial To Parallel : allblocks_alteradspbuilder2/Serial To Parallel  BusType=Unsigned Integer  bwl=12  bwr=0  msbfirsttext=LSB First  msbfirst=0  use_ena=on  use_sclr=on
  Shift by Two : allblocks_alteradspbuilder2/Bus Conversion  BusType=Signed Integer  ibwl=20  ibwr=0  bwl=19  bwr=0  bitToConnectToOutputLSB=1  round=off  saturate=off  pipeline_display=0
  Sync Delay : allblocks_alteradspbuilder2/Memory Delay  BusType=Inferred  bwl=8  bwr=0  pipeline=17  pipeline_display=17  ram_type=AUTO  use_ena=off  use_sclr=off  allowFloatingPointOverride=on  logOutputs=off  logFile=/data/akarapet/qshell_linux64_test/p4/dsp_builder/dsp_builder2/Documentation/DesignExamples/Demos/Filters/FilteringLab/Stap/tb_StFilteringLab/StFilteringLab_LowPass%5FSerialFilter_Scaling+Accumulator_Sync+Delay.fixedpointlog
  Sync Delay2 : allblocks_alteradspbuilder2/Delay  pipeline=1  pipeline_display=1  ClockPhase=1  use_ena=off  use_sclr=off  allowFloatingPointOverride=on  logOutputs=off  logFile=/data/akarapet/qshell_linux64_test/p4/dsp_builder/dsp_builder2/Documentation/DesignExamples/Demos/Filters/FilteringLab/Stap/tb_StFilteringLab/StFilteringLab_LowPass%5FSerialFilter_Scaling+Accumulator_Sync+Delay2.fixedpointlog  use_init=off  reset_value=1
  Terminator : Terminator
  VCC1 : allblocks_alteradspbuilder2/VCC  SpecifyClock=off
  VCC2 : allblocks_alteradspbuilder2/VCC  SpecifyClock=off
  Out[17:0] : Outport
  wires:
  BusBuild/1 -> Inverse Last Partial Product/2
  Output Resolution Area of Interrest/1 -> Delay4/1
  Sync Delay2/1 -> [Sync]
  Pipeline  Delay/1 -> Inverse Last Partial Product/1
  Inverse Last Partial Product/1 -> Adder/2
  In[18:0]/1 -> Pipeline  Delay/1
  Sync Delay/1 -> Adder/3, BusBuild/1, BusBuild/2, Sync Delay2/1
  Adder/2 -> Delay/1, ExtractBit/1
  VCC2/1 -> Adder/4
  [Sync] -> Reset On Last Partial Product/1
  [FeedBack] -> Reset On Last Partial Product/2
  clr/1 -> Sync Delay/1
  GND2/1 -> Reset On Last Partial Product/3
  Reset On Last Partial Product/1 -> Adder/1
  ExtractBit/1 -> Serial To Parallel/1
  BusConcatenation/1 -> Output Resolution Area of Interrest/1
  GND1/1 -> Delay4/3
  GND/1 -> Serial To Parallel/3
  Serial To Parallel/1 -> BusConcatenation/2
  VCC1/1 -> Serial To Parallel/2
  Shift by Two/1 -> [FeedBack], BusConcatenation/1
  Delay/1 -> Shift by Two/1
  Delay4/1 -> Out[17:0]/1
  [Sync] -> Delay4/2
  Adder/1 -> Terminator/1
